simulink model "ddmr_model_ush"  (R2023b)
settings: Solver=VariableStepAuto  StartTime=0.0  StopTime=10.0  RelTol=1e-3
values from neighbouring files (symbols this model uses):
  alpha_k = constantes(14)    [calculaMatrizesModelo.m]    (also in integracaoNumerica.m = c(12); simulaModeloSimulink.m; simulaTrajetoriaSimulink.m)
  alpha_s = constantes(13)    [calculaMatrizesModelo.m]    (also in integracaoNumerica.m = c(11); simulaModeloSimulink.m; simulaTrajetoriaSimulink.m)
  b = constantes(7)    [calculaMatrizesModelo.m]    (also in integracaoNumerica.m = c(3); simulaModeloSimulink.m; simulaTrajetoriaSimulink.m)
  d = constantes(5)    [calculaMatrizesModelo.m]    (also in simulaModeloSimulink.m; simulaTrajetoriaSimulink.m)
  f_k = constantes(12)    [calculaMatrizesModelo.m]    (also in simulaModeloSimulink.m; simulaTrajetoriaSimulink.m)
  f_s = constantes(11)    [calculaMatrizesModelo.m]    (also in simulaModeloSimulink.m; simulaTrajetoriaSimulink.m)
  I_t = I_c + 2*m_w*L^2 + 2*I_w + m_c*d^2    [calculaMatrizesModelo.m]    (also in simulaModeloSimulink.m; simulaTrajetoriaSimulink.m)
  K_ce = constantes(8)    [calculaMatrizesModelo.m]    (also in simulaModeloSimulink.m; simulaTrajetoriaSimulink.m)
  k_i = constantes(15)    [calculaMatrizesModelo.m]    (also in simulaModeloSimulink.m; simulaTrajetoriaSimulink.m)
  k_p = constantes(16)    [calculaMatrizesModelo.m]    (also in simulaModeloSimulink.m; simulaTrajetoriaSimulink.m)
  K_t = constantes(9)    [calculaMatrizesModelo.m]    (also in simulaModeloSimulink.m; simulaTrajetoriaSimulink.m)
  L = constantes(2)    [calculaMatrizesModelo.m]    (also in integracaoNumerica.m = c(2); simulaModeloSimulink.m; simulaTrajetoriaSimulink.m)
  m = m_c + 2*m_w    [calculaMatrizesModelo.m]    (also in integracaoNumerica.m = mc + 2*mw; simulaModeloSimulink.m; simulaTrajetoriaSimulink.m)
  N = constantes(6)    [calculaMatrizesModelo.m]    (also in integracaoNumerica.m = 1; simulaModeloSimulink.m; simulaTrajetoriaSimulink.m)
  R = 0.034    [calculaErros.m]    (also in calculaMatrizesModelo.m = constantes(1); integracaoNumerica.m = c(1); plotTrajetoria.m = 0.175; simulaModeloSimulink.m = constantes(1))
  R_a = constantes(10)    [calculaMatrizesModelo.m]    (also in simulaModeloSimulink.m; simulaTrajetoriaSimulink.m)
libraries: simulink x1
settings Model: Creator=Gabriel Sousa  LastModifiedBy=Gabriel Sousa

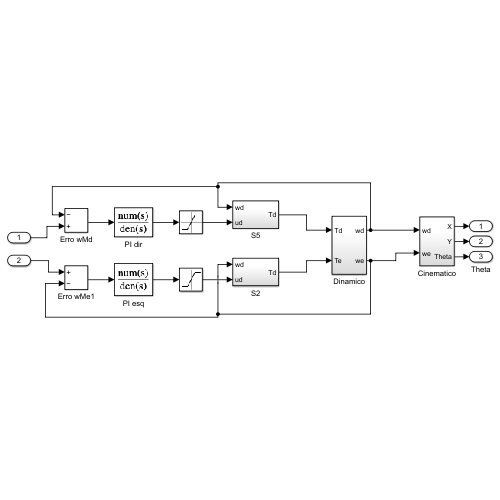
[thumbnail: Simulink's stored preview of the top-level diagram]
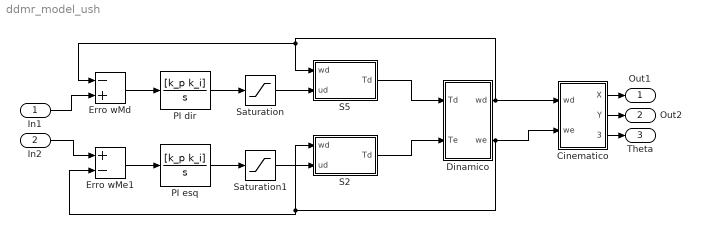
== system ddmr_model_ush ==
  In1 : Inport
  In2 : Inport  Port=2
  Cinematico : Subsystem
  Dinamico : Subsystem
  Erro wMd : Sum  Inputs=-+
  Erro wMe1 : Sum  Inputs=+-
  PI dir : TransferFcn  Numerator=[k_p k_i]  Denominator=[1 0]
  PI esq : TransferFcn  Numerator=[k_p k_i]  Denominator=[1 0]
  S2 : Subsystem
  S5 : Subsystem
  Saturation : Saturate  UpperLimit=12  LowerLimit=-12
  Saturation1 : Saturate  UpperLimit=12  LowerLimit=-12
  Out1 : Outport
  Out2 : Outport  Port=2
  Theta : Outport  Port=3
  wires:
  Dinamico/1(wd) -> Erro wMd/1, S5/1(wd), Cinematico/1(wd)
  Saturation/1 -> S5/2(ud)
  Dinamico/2(we) -> S2/1(wd), Erro wMe1/2, Cinematico/2(we)
  PI dir/1 -> Saturation/1
  Erro wMd/1 -> PI dir/1
  In2/1 -> Erro wMe1/1
  PI esq/1 -> Saturation1/1
  In1/1 -> Erro wMd/2
  Saturation1/1 -> S2/2(ud)
  S5/1(Td) -> Dinamico/1(Td)
  Erro wMe1/1 -> PI esq/1
  S2/1(Td) -> Dinamico/2(Te)
  Cinematico/1(X) -> Out1/1
  Cinematico/2(Y) -> Out2/1
  Cinematico/3(Theta) -> Theta/1

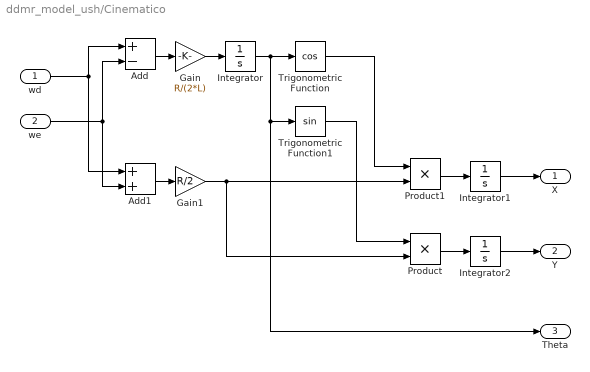
== system ddmr_model_ush/Cinematico ==
  wd : Inport
  we : Inport  Port=2
  Add : Sum  Inputs=+-
  Add1 : Sum
  Gain : Gain  Gain=R/(2*L)
  Gain1 : Gain  Gain=R/2
  Integrator : Integrator
  Integrator1 : Integrator
  Integrator2 : Integrator
  Product : Product
  Product1 : Product
  Trigonometric Function : Trigonometry  Operator=cos
  Trigonometric Function1 : Trigonometry
  X : Outport  VectorParamsAs1DForOutWhenUnconnected=off
  Y : Outport  Port=2  VectorParamsAs1DForOutWhenUnconnected=off
  Theta : Outport  Port=3  VectorParamsAs1DForOutWhenUnconnected=off
  wires:
  wd/1 -> Add/1, Add1/1
  we/1 -> Add/2, Add1/2
  Add/1 -> Gain/1
  Gain/1 -> Integrator/1
  Integrator/1 -> Theta/1, Trigonometric Function1/1, Trigonometric Function/1
  Add1/1 -> Gain1/1
  Gain1/1 -> Product/2, Product1/2
  Trigonometric Function/1 -> Product1/1
  Trigonometric Function1/1 -> Product/1
  Product/1 -> Integrator2/1
  Product1/1 -> Integrator1/1
  Integrator1/1 -> X/1
  Integrator2/1 -> Y/1

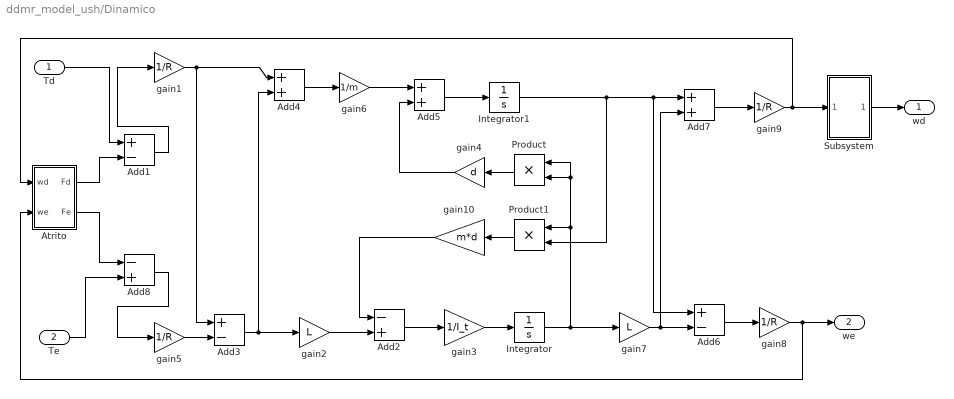
== system ddmr_model_ush/Dinamico ==
  Td : Inport
  Te : Inport  Port=2
  Add1 : Sum  Inputs=+-
  Add2 : Sum  Inputs=-+
  Add3 : Sum  Inputs=+-
  Add4 : Sum
  Add5 : Sum
  Add6 : Sum  Inputs=+-
  Add7 : Sum
  Add8 : Sum  Inputs=-+
  Atrito : Subsystem
  Integrator : Integrator
  Integrator1 : Integrator
  Product : Product
  Product1 : Product
  Subsystem : Subsystem
  gain{1,5,8..9} (4 alike) : Gain  Gain=1/R
  gain10 : Gain  Gain=m*d
  gain2 : Gain  Gain=L
  gain3 : Gain  Gain=1/I_t
  gain4 : Gain  Gain=d
  gain6 : Gain  Gain=1/m
  gain7 : Gain  Gain=L
  wd : Outport  VectorParamsAs1DForOutWhenUnconnected=off
  we : Outport  Port=2  VectorParamsAs1DForOutWhenUnconnected=off
  wires:
  gain5/1 -> Add3/2
  gain1/1 -> Add3/1, Add4/1
  Add3/1 -> Add4/2, gain2/1
  Add4/1 -> gain6/1
  gain6/1 -> Add5/1
  gain2/1 -> Add2/2
  Add2/1 -> gain3/1
  gain3/1 -> Integrator/1
  Integrator/1 -> Product1/1, Product/2, Product/1, gain7/1
  gain7/1 -> Add7/2, Add6/2
  Add6/1 -> gain8/1
  Add5/1 -> Integrator1/1
  Integrator1/1 -> Product1/2, Add6/1, Add7/1
  Add7/1 -> gain9/1
  gain4/1 -> Add5/2
  Product/1 -> gain4/1
  Product1/1 -> gain10/1
  gain10/1 -> Add2/1
  Td/1 -> Add1/1
  Te/1 -> Add8/2
  gain8/1 -> Atrito/2(we), we/1
  Add1/1 -> gain1/1
  Atrito/1(Fd) -> Add1/2
  Atrito/2(Fe) -> Add8/1
  Add8/1 -> gain5/1
  gain9/1 -> Subsystem/1(In1), Atrito/1(wd)
  Subsystem/1(Out1) -> wd/1

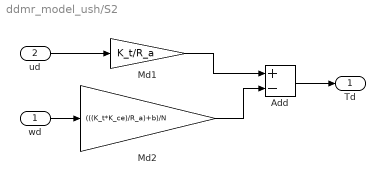
== system ddmr_model_ush/S2 ==
  wd : Inport
  ud : Inport  Port=2
  Add : Sum  Inputs=+-
  Md1 : Gain  Gain=K_t/R_a
  Md2 : Gain  Gain=(((K_t*K_ce)/R_a)+b)/N
  Td : Outport  VectorParamsAs1DForOutWhenUnconnected=off
  wires:
  Md1/1 -> Add/1
  Md2/1 -> Add/2
  wd/1 -> Md2/1
  ud/1 -> Md1/1
  Add/1 -> Td/1

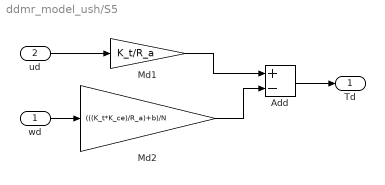
== system ddmr_model_ush/S5 ==
  wd : Inport
  ud : Inport  Port=2
  Add : Sum  Inputs=+-
  Md1 : Gain  Gain=K_t/R_a
  Md2 : Gain  Gain=(((K_t*K_ce)/R_a)+b)/N
  Td : Outport  VectorParamsAs1DForOutWhenUnconnected=off
  wires:
  Md1/1 -> Add/1
  Md2/1 -> Add/2
  wd/1 -> Md2/1
  ud/1 -> Md1/1
  Add/1 -> Td/1

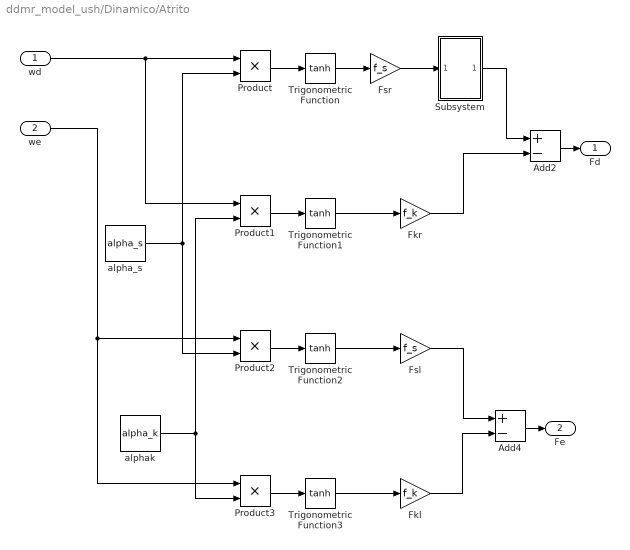
== system ddmr_model_ush/Dinamico/Atrito ==
  wd : Inport
  we : Inport  Port=2
  Add2 : Sum  Inputs=+-
  Add4 : Sum  Inputs=+-
  Fkl : Gain  Gain=f_k
  Fkr : Gain  Gain=f_k
  Fsl : Gain  Gain=f_s
  Fsr : Gain  Gain=f_s
  Product{,1..3} (4 alike) : Product
  Subsystem : Subsystem
  Trigonometric Function{,1..3} (4 alike) : Trigonometry  Operator=tanh
  alpha_s : Constant  Value=alpha_s
  alphak : Constant  Value=alpha_k
  Fd : Outport  VectorParamsAs1DForOutWhenUnconnected=off
  Fe : Outport  Port=2  VectorParamsAs1DForOutWhenUnconnected=off
  wires:
  we/1 -> Product2/1, Product3/1
  wd/1 -> Product/1, Product1/1
  Fsl/1 -> Add4/1
  Trigonometric Function2/1 -> Fsl/1
  Trigonometric Function/1 -> Fsr/1
  Fkl/1 -> Add4/2
  Trigonometric Function3/1 -> Fkl/1
  Trigonometric Function1/1 -> Fkr/1
  Fkr/1 -> Add2/2
  alphak/1 -> Product1/2, Product3/2
  Product3/1 -> Trigonometric Function3/1
  Product2/1 -> Trigonometric Function2/1
  alpha_s/1 -> Product/2, Product2/2
  Add4/1 -> Fe/1
  Add2/1 -> Fd/1
  Product1/1 -> Trigonometric Function1/1
  Product/1 -> Trigonometric Function/1
  Fsr/1 -> Subsystem/1(In1)
  Subsystem/1(Out1) -> Add2/1

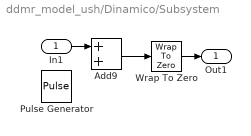
== system ddmr_model_ush/Dinamico/Subsystem ==
  In1 : Inport
  Add9 : Sum
  Pulse Generator : DiscretePulseGenerator  PulseType=Time based  Amplitude=100  Period=200  PulseWidth=0.8  PhaseDelay=45
  Wrap To Zero : simulink/Discontinuities/Wrap To Zero  Threshold=80
  Out1 : Outport  VectorParamsAs1DForOutWhenUnconnected=off
  wires:
  Add9/1 -> Wrap To Zero/1
  Wrap To Zero/1 -> Out1/1
  In1/1 -> Add9/1

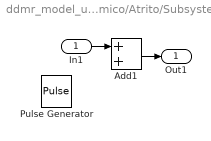
== system ddmr_model_ush/Dinamico/Atrito/Subsystem ==
  In1 : Inport
  Add1 : Sum
  Pulse Generator : DiscretePulseGenerator  PulseType=Time based  Amplitude=0.075  Period=200  PulseWidth=2.5  PhaseDelay=220
  Out1 : Outport  VectorParamsAs1DForOutWhenUnconnected=off
  wires:
  Add1/1 -> Out1/1
  In1/1 -> Add1/1
